simulink model "TemperCelsius2Fahrenheit"  (R2022b)
settings: Solver=VariableStepAuto  StartTime=0.0  StopTime=10.0  RelTol=1e-3
libraries: simulink x1
settings Model: Creator=Andrey  LastModifiedBy=Andrey

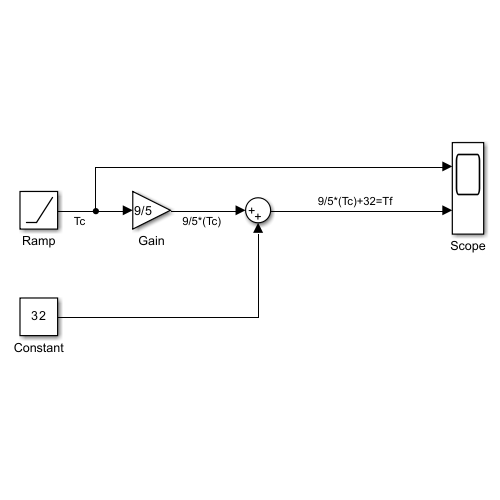
[thumbnail: Simulink's stored preview of the top-level diagram]
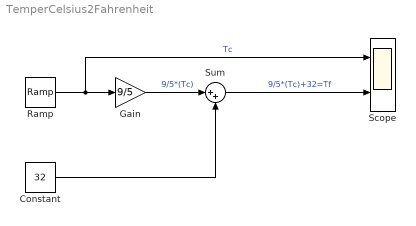
== system TemperCelsius2Fahrenheit ==
  Constant : Constant  Value=32
  Gain : Gain  Gain=9/5
  Ramp : simulink/Sources/Ramp  slope=1  start=0  InitialOutput=0
  Scope : Scope  NumInputPorts=2
  Sum : Sum  Inputs=|++
  wires:
  Ramp/1 -> Scope/1, Gain/1  "Tc"
  Gain/1 -> Sum/1  "9/5*(Tc)"
  Constant/1 -> Sum/2
  Sum/1 -> Scope/2  "9/5*(Tc)+32=Tf"
